simulink model "uuvSim_simple"  (R2017a)
settings: Solver=ode4  StartTime=0.0  StopTime=10.0  FixedStep=mdl.tStep  RelTol=1e-3
undefined symbols (not defined in the file): ics, rov, tau, v_c
settings Model: Creator=e_anderlini  LastModifiedBy=e_anderlini

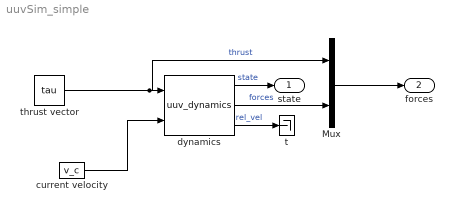
== system uuvSim_simple ==
  Mux : Mux  Inputs=[6,18]
  current velocity : Constant  Value=v_c
  dynamics : S-Function  FunctionName=uuv_dynamics  Parameters=rov.weight,rov.buoyancy,rov.G,rov.B,ics,rov.inv_mass',rov.M_A',rov.M_RB',rov.D_L',rov.D_q'  SFunctionDeploymentMode=off  EnableBusSupport=off
  t : Terminator
  thrust vector : Constant  Value=tau
  state : Outport
  forces : Outport  Port=2
  wires:
  dynamics/1 -> state/1  "state"
  Mux/1 -> forces/1
  dynamics/2 -> Mux/2  "forces"
  thrust vector/1 -> Mux/1, dynamics/1  "thrust"
  current velocity/1 -> dynamics/2
  dynamics/3 -> t/1  "rel_vel"
